simulink model "SimulinkCavalca"  (Simulink 8.2)
settings: Solver=ode4  SolverMode=SingleTasking  StartTime=0.0  StopTime=25  FixedStep=0.01  RelTol=1e-3
InitFcn:
  | Main;
undefined symbols (not defined in the file): A1, B1, C, Cstate, Dstate, T, xk0, Ymax
settings Model: Creator=Kawakami  LastModifiedBy=Eduardo
settings DataIOCC: LimitDataPoints=off  SaveOutput=off  SaveTime=off  TimeSaveName=t  SignalLoggingName=sigsOut
settings OptimizationCC: BooleanDataType=off
settings DebuggingCC: SaveWithParameterizedLinksMsg=none  SignalResolutionControl=TryResolveAllWithWarning  SolverPrmCheckMsg=none  MultiTaskDSMMsg=warning  MultiTaskCondExecSysMsg=none
settings HardwareCC: TargetUnknown=on
settings RTWCC: IncludeERTFirstTime=on

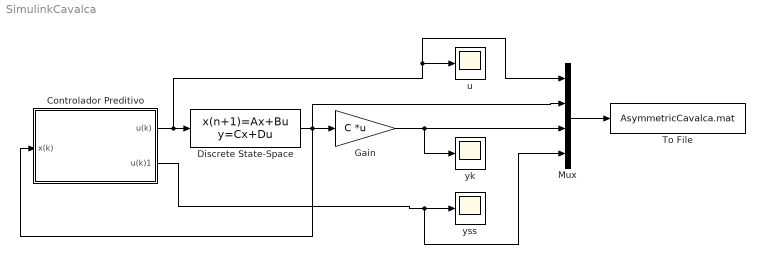
== system SimulinkCavalca ==
  "Controlador Preditivo  " : Subsystem
  Discrete State-Space : DiscreteStateSpace  A=A1  B=B1  C=Cstate  D=Dstate  X0=xk0  SampleTime=T
  Gain : Gain  Gain=C  Multiplication=Matrix(K*u)  SampleTime=T
  Mux : Mux
  To File : ToFile  Filename=AsymmetricCavalca.mat  MatrixName=Cavalca  SampleTime=T
  u : Scope
      settings: TimeRange=10  YMin=-3e-06  YMax=1.1e-05
  yk : Scope
      settings: YMin=-1.25  YMax=2.25
  yss : Scope
      settings: YMin=-1.25  YMax=2.25  SaveName=ScopeData2
  wires:
  "Controlador Preditivo  "/1(u(k)) -> Mux/1, u/1, Discrete State-Space/1
  Discrete State-Space/1 -> Mux/2, Gain/1, "Controlador Preditivo  "/1(x(k))
  Gain/1 -> yk/1, Mux/3
  Mux/1 -> To File/1
  "Controlador Preditivo  "/2(u(k)1) -> Mux/4, yss/1

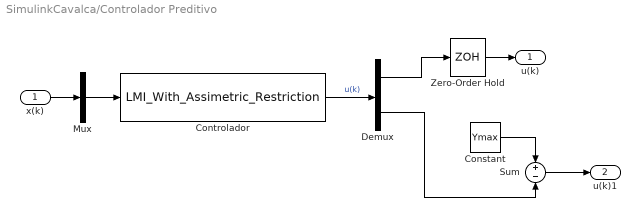
== system SimulinkCavalca/Controlador Preditivo   ==
  x(k) : Inport
  Constant : Constant  Value=Ymax  SampleTime=T
  Controlador : S-Function  FunctionName=LMI_With_Assimetric_Restriction  Parameters=A, B, C, Smeio, Rmeio, Umax, imax, Qsol, xref, yb, T  EnableBusSupport=off
  Demux : Demux  Outputs=2
  Mux : Mux  Inputs=1
  Sum : Sum  Inputs=+|-  SampleTime=T
  Zero-Order Hold : ZeroOrderHold  SampleTime=T
  u(k) : Outport
  u(k)1 : Outport  Port=2
  wires:
  Zero-Order Hold/1 -> u(k)/1
  Controlador/1 -> Demux/1  "u(k)"
  Mux/1 -> Controlador/1
  x(k)/1 -> Mux/1
  Demux/1 -> Zero-Order Hold/1
  Constant/1 -> Sum/1
  Demux/2 -> Sum/2
  Sum/1 -> u(k)1/1
